simulink model "final"  (R2019b)
settings: Solver=VariableStepAuto  StartTime=0.0  StopTime=70  RelTol=1e-3
undefined symbols (not defined in the file): DiscIntNeverNeededParam, sigbuilder_block
libraries: simulink x2
settings Model: Creator=dayam1  LastModifiedBy=prachurjyas1
settings OptimizationCC: DefaultParameterBehavior=Inlined  EnhancedBackFolding=on  PassReuseOutputArgsThreshold=0  OptimizeBlockOrder=speed  DifferentSizesBufferReuse=on  OptimizationCustomize=off
settings DebuggingCC: SignalInfNanChecking=warning  ParameterTunabilityLossMsg=error  UniqueDataStoreMsg=warning  StrictBusMsg=ErrorOnBusTreatedAsVector
settings SFSimCC: MATLABDynamicMemAlloc=off
settings RTWCC: Description=Generic Real-Time Target  GenerateReport=on  LaunchReport=on
settings CodeAppCC: ForceParamTrailComments=on  OperatorAnnotations=on
settings ConfigComp: CovMetricSettings=dcmwe

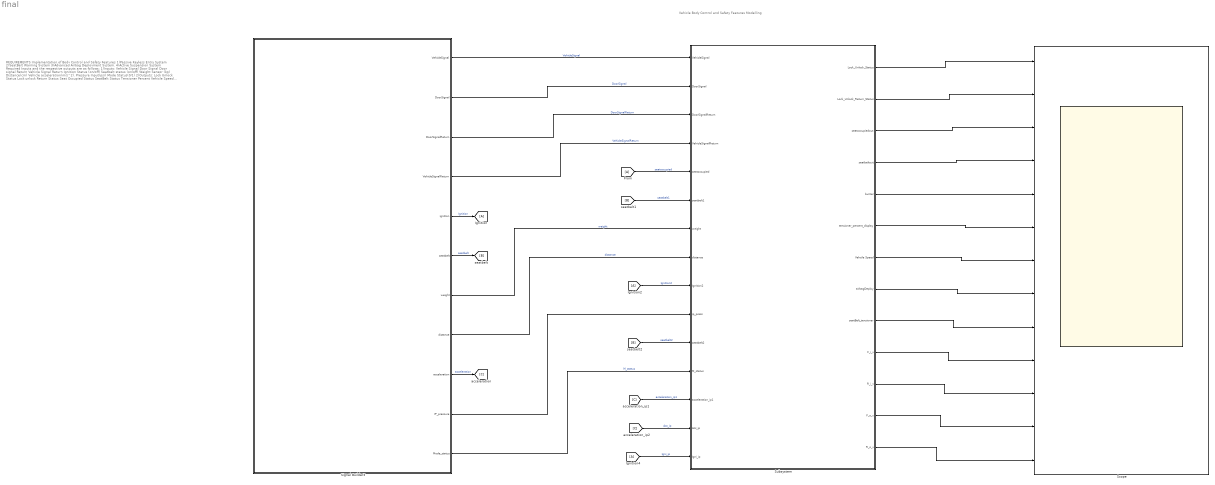
== system final ==
  note: REQUIREMENTS
      |
      | Implementation of Body Control and Safety Features
      | 1)Passive Keyless Entry System
      | 2)SeatBelt Warning System
      | 3)Advanced Airbag Deployment System.
      | 4)Active Suspension System
      |
      | Required Inputs and the respective outputs are as follows:
      | 1)Inputs: Vehicle Signal
      | Door Signal
      | Door signal Return
      | Vehicle Signal Return
      | Ignition Status (on/off)
      | Seatbelt status (on/off)
      | Weight Sensor (kg)
      | Distance(cm)
      | Vehicle acceleration(m/s^2).
      | Pressure Input(psi)
      | Mode Status(0/1)
      |
      | 2)Outputs:
      | Lock Unlock Status
      | Lock unlock Return Status
      | Seat Occupied Status
      | SeatBelt Status
      | Tensioner Percent
      | Vehicle Speed
      | Airbag Deployment
      | Seatbelt tensioner status
      | Steering Status
  note: Vehicle Body Control and Safety Features Modelling
  Scope : Scope  NumInputPorts=13
  Signal Builder3 : Subsystem  Tag=STV Subsys  LoadFcn=sigbuilder_block('load');  StartFcn=sigbuilder_block('start');  StopFcn=sigbuilder_block('stop');  ClipboardFcn=sigbuilder_block('clipboard');  mask(Sigbuilder block){tuvar=[0:10]}
      mask help: Create and generate interchangeable groups of signals whose waveforms are piecewise linear.
      mask init:
      | if ~strcmp(get_param(bdroot(gcbh),'SimulationStatus'),'stopped') tuvar = sigbuilder_block('maskInit'); end
      settings: CopyFcn=sigbuilder_block('copy');  DeleteFcn=sigbuilder_block('delete');  ModelCloseFcn=sigbuilder_block('modelClose');  PreSaveFcn=sigbuilder_block('preSave');  PauseFcn=sigbuilder_block('pause')  ContinueFcn=sigbuilder_block('continue')  NameChangeFcn=sigbuilder_block('namechange');  OpenFcn=sigbuilder_block('open',[6 30 1012.5 447.75 ]);  CloseFcn=sigbuilder_block('close');
      mask Display: plot(0, 0, 100, 100,[2, 2, 32, 32, 2], [68, 8, 8, 68, 68],[32, 2], [38, 38], [32, 19, 2],[53, 60, 44], [32, 17, 17, 2],[16, 16, 31, 31]);txt = getActiveGroup(gcbh);text(2, 100, txt,'verticalAlignment', 'top');
  Subsystem : Subsystem
  wires:
  Signal Builder3/6(seatbelt) -> [B]  "seatbelt"
  Signal Builder3/9(acceleration) -> [C]  "acceleration"
  Signal Builder3/5(ignition) -> [A]  "Ignition"
  [A] -> Subsystem/15(Igni_ip)  "Igni_ip"
  Signal Builder3/1(VehicleSignal) -> Subsystem/1(VehicleSignal)  "VehicleSignal"
  Signal Builder3/2(DoorSignal) -> Subsystem/2(DoorSignal)  "DoorSignal"
  Signal Builder3/3(DoorSignalReturn) -> Subsystem/3(DoorSignalReturn)  "DoorSignalReturn"
  Signal Builder3/4(VehicleSignalReturn) -> Subsystem/4(VehicleSignalReturn)  "VehicleSignalReturn"
  [A] -> Subsystem/5(seatoccupied)  "seatoccupied"
  [B] -> Subsystem/6(seatbelt1)  "seatbelt1"
  Signal Builder3/7(weight) -> Subsystem/7(weight)  "weight"
  Signal Builder3/8(distance) -> Subsystem/8(distance)  "distance"
  [A] -> Subsystem/9(Ignition2)  "Ignition2"
  Signal Builder3/10(IP_pressure) -> Subsystem/10(ip_press)
  [B] -> Subsystem/11(seatbelt2)  "seatbelt2"
  Signal Builder3/11(Mode_status) -> Subsystem/12(M_status)  "M_status"
  [C] -> Subsystem/13(acceleration_ip1)  "acceleration_ip1"
  [C] -> Subsystem/14(Acc_ip)  "Acc_ip"
  Subsystem/1("Lock_Unlock_Status ") -> Scope/1
  Subsystem/2(Lock_Unlock_Return_Status) -> Scope/2
  Subsystem/3(seatoccupiedout) -> Scope/3
  Subsystem/4(seatbeltout) -> Scope/4
  Subsystem/5(buzzer) -> Scope/5
  Subsystem/6(tensioner_percent_display) -> Scope/6
  Subsystem/7(Vehcile Speed) -> Scope/7
  Subsystem/8(airbagDeploy) -> Scope/8
  Subsystem/9(seatBelt_tensioner) -> Scope/9
  Subsystem/10(F_i_v) -> Scope/10
  Subsystem/11(R_i_v) -> Scope/11
  Subsystem/12(F_o_v) -> Scope/12
  Subsystem/13(R_o_v) -> Scope/13

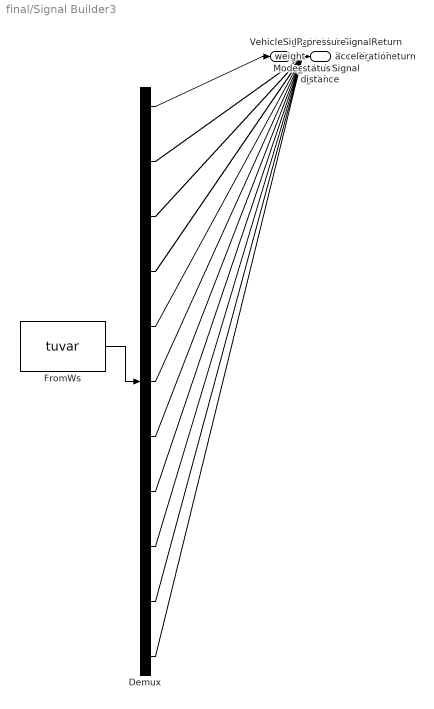
== system final/Signal Builder3 ==
  Demux : Demux  Tag=STV Demux  Outputs=11
  FromWs : FromWorkspace  Tag=STV FromWs  VariableName=tuvar  SampleTime=0
      SigBuilderData=|
      | common.afterFinalStr = 'Extrapolate'
      | common.sampleTime = 0
      | dataSet.timeRange = [0 69]
      | dataSet.name = 'Signal_input'
      | sbobj.Groups.Name = 'Signal_input'
      | sbobj.Groups.Signals(1).Name = 'VehicleSignal'
      | sbobj.Groups.Signals(1).XData = [0 2 10.18 10.18 10.4 10.4 18.94 18.94 20 69]
      | sbobj.Groups.Signals(1).YData = [100 190 558.1 500 500 568 952.3 140 180 180]
      | sbobj.Groups.Signals(2).Name = 'DoorSignal'
      | sbobj.Groups.Signals(2).XData = [0 2 12.26 12.36 12.8 12.8 19.04 19.04 20 69]
      | sbobj.Groups.Signals(2).YData = [0 20 122.6 120 120 128 190.4 -20 -10 -10]
      | sbobj.Groups.Signals(3).Name = 'DoorSignalReturn'
      | sbobj.Groups.Signals(3).XData = [0 18 69]
      | sbobj.Groups.Signals(3).YData = [199.6 0 0]
      | sbobj.Groups.Signals(4).Name = 'VehicleSignalReturn'
      | sbobj.Groups.Signals(4).XData = [0 18 69]
      | sbobj.Groups.Signals(4).YData = [1000 100 100]
      | sbobj.Groups.Signals(5).Name = 'ignition'
      | sbobj.Groups.Signals(5).XData = [0 1 2 3 4 5 6 7 7 8 9 9 10 11 11 12 13 13 14 15 16 17 18 19 20 21 22 23 24 25 26 27 28 29 30 31 31.5 31.9 32.3 32.7 33.1 33.5 33.9 34.3 34.7 35.1 35.5 35.9 36.3 36.7 37.1 37.5 37.9 38.3 39 40 41 42 43 44 45 46 47 48 49 50 51 52 53 54 55 56 57 58 59 60 61 62 63 64 65 66 67 68 69]
      | sbobj.Groups.Signals(5).YData = [0 0 0 1 1 1 1 1 0 0 0 1 1 1 0 0 0 1 1 1 1 1 1 1 1 1 1 1 1 1 1 1 1 1 1 1 0 0 0 0 0 0 0 0 0 0 0 0 0 0 0 0 0 0 0 1 1 1 1 1 1 0 1 1 1 1 0 1 1 0 1 1 1 0 1 1 1 1 1 1 1 1 1 1 0]
      | sbobj.Groups.Signals(6).Name = 'seatbelt'
      | sbobj.Groups.Signals(6).XData = [0 1 2 3 3 4 4 5 6 7 7 8 9 10 11 12 13 13 14 15 16 17 18 18 19 20 21 22 23 24 25 26 27 28 29 30 31 31 31.5 31.9 32.3 32.7 33.1 33.5 33.9 34.3 34.7 35.1 35.5 35.9 36.3 36.7 37.1 37.5 37.9 38.3 39 40 40 41 42 43 44 45 46 47 48 49 50 50 51 52 53 54 55 56 57 58 59 60 60 61 62 63 64 65 66 67 68 69]
      | sbobj.Groups.Signals(6).YData = [0 0 0 0 1 1 0 0 0 0 1 1 1 1 1 1 1 0 0 0 0 0 0 1 1 1 1 1 1 1 1 1 1 1 1 1 1 0 0 0 1 1 1 1 1 1 1 1 1 1 1 1 1 1 1 1 1 1 0 0 1 1 1 1 1 1 1 1 1 0 0 1 1 1 1 1 1 1 1 1 0 0 1 1 1 1 1 1 1 1]
      | sbobj.Groups.Signals(7).Name = 'weight'
      | sbobj.Groups.Signals(7).XData = [0 1 1 2 2 3 3 4 4 5 5 6 6 7 7 8 8 9 9 10 10 11 11 12 12 13 13 14 14 15 15 16 16 17 17 18 18 19 19 20 20 21 21 22 23 24 24 25 25 26 26 27 27 28 28 29 29 30 30 31 31 31.5 31.9 32.3 32.7 33.1 33.5 33.9 34.3 34.7 35.1 35.5 35.9 36.3 36.7 37.1 37.5 37.9 38.3 39 40 41 42 43 44 45 46 47 48 49 50 51 52 52 53 53 54 55 56 57 58 58 59 60 60 61 62 63 63 64 64 65 65 66 66 67 67 68 68 69]
      | sbobj.Groups.Signals(7).YData = [78 78 68 66 55 55 87 87 43 43 30 30 20 20 10 10 70 70 88 88 99 99 66 66 54 54 34 34 44 44 89 89 86 86 10 10 54 54 44 44 99 99 75 106 106 50 25 25 33 33 26 26 57 57 78 78 57 57 78 78 86 10 10 54 54 44 44 99 99 75 106 106 106 106 50 25 25 33 33 66 55 87 43 30 20 10 70 88 99 66 54 34 44 78 78 86 10 54 44 99 75 106 106 106 50 25 33 66 78 86 10 10 54 54 44 44 99 99 75 106]
      | sbobj.Groups.Signals(8).Name = 'distance'
      | sbobj.Groups.Signals(8).XData = [0 1 2 3 4 5 6 7 8 9 10 11 12 13 14 15 16 17 18 19 20 21 22 23 24 25 26 27 28 29 30 31 31 31.5 31.9 32.3 32.7 33.1 33.5 33.9 34.3 34.7 35.1 35.5 35.9 36.3 36.7 37.1 37.5 37.9 38.3 39 40 40 41 41 42 42 43 43 44 44 45 45 46 46 47 47 48 48 49 49 50 51 52 53 54 55 56 57 58 59 60 60 61 61 62 62 63 63 64 64 65 65 66 66 67 67 68 68 69]
      | sbobj.Groups.Signals(8).YData = [21 22 24 10 18 23 29 50 23 16 13 21 22 19 14 24 15 19 11 22 17 22 24 10 18 23 29 50 23 50 23 23 19 19 11 11 22 22 17 17 22 22 24 24 10 10 18 18 23 23 29 17 17 22 22 24 24 10 10 18 18 23 23 29 29 50 50 23 23 50 50 23 23 19 11 22 17 22 24 10 18 23 29 17 17 22 22 24 24 10 10 18 18 23 23 29 29 50 50 23 23]
      | sbobj.Groups.Signals(9).Name = 'acceleration'
      | sbobj.Groups.Signals(9).XData = [0 1 2 3 4 5 6 7 8 9 10 11 12 13 14 15 16 17 18 19 20 21 22 23 24 25 26 27 28 29 30 31 31 31.5 31.9 32.3 32.7 33.1 33.5 33.9 34.3 34.7 35.1 35.5 35.9 36.3 36.7 37.1 37.5 37.9 38.3 39 40 41 42 43 44 45 46 47 48 49 50 51 52 53 54 55 56 57 58 59 60 61 62 63 64 65 66 67 68 69]
      | sbobj.Groups.Signals(9).YData = [9 12 45 54 67 12 47 34 67 23 89 23 52 9 76 13 67 34 90 28 49 12 45 54 67 12 47 34 67 34 67 67 34 34 90 90 90 90 90 90 90 90 90 45 54 54 67 67 12 12 47 12 45 54 67 20 50 34 67 23 89 23 52 76 50 13 67 45 14 88 49 42 45 24 67 12 99 34 67 50 99 9]
      | sbobj.Groups.Signals(10).Name = 'IP_pressure'
      | sbobj.Groups.Signals(10).XData = [0 1 2 3 4 5 6 7 8 9 10 11 12 13 14 15 16 17 18 19 20 21 22 23 24 25 26 27 28 29 30 31 31 31.5 31.9 32.3 32.7 33.1 33.5 33.9 34.3 34.7 35.1 35.5 35.9 36.3 36.7 37.1 37.5 37.9 38.3 39 40 41 42 43 44 45 46 47 48 49 50 51 52 53 54 55 56 57 58 59 60 61 62 63 64 65 66 67 68 69]
      | sbobj.Groups.Signals(10).YData = [-100 -80 60 45 65 100 76 23 98 45 119 102 99 66 34 56 22 97 67 9 78 -80 60 45 65 100 76 23 98 23 0 0 97 97 67 67 9 9 78 78 -80 -80 60 60 45 45 65 65 100 100 76 -50 -10 10 30 50 50 100 110 100 40 80 140 50 50 15 17 100 100 100 88 100 50 50 44 66 50 50 100 100 50 -100]
      | sbobj.Groups.Signals(11).Name = 'Mode_status'
      | sbobj.Groups.Signals(11).XData = [0 1 2 2 3 4 5 6 7 7 8 9 9 10 11 11 12 13 13 14 15 16 17 18 19 20 21 22 22 23 24 25 26 27 27 28 29 30 31 31.5 31.9 32.3 32.7 33.1 33.5 33.9 34.3 34.7 35.1 35.5 35.9 36.3 36.7 37.1 37.5 37.9 38.3 39 40 41 42 43 44 45 46 47 48 49 50 51 52 53 54 55 56 57 58 59 60 61 62 63 64 65 66 67 68 69]
      | sbobj.Groups.Signals(11).YData = [0 0 0 1 1 1 1 1 1 0 0 0 1 1 1 0 0 0 1 1 1 1 1 1 1 1 0 0 1 1 1 1 1 1 0 0 1 1 1 1 1 1 1 1 1 1 0 0 0 1 1 1 1 1 1 1 1 0 1 1 1 0 0 1 1 1 0 0 0 0 0 0 0 1 1 1 0 1 0 0 0 0 0 0 1 1 0 0]
      | sbobj.Groups.TimeRange = [0 69]
  VehicleSignal : Outport  Tag=STV Outport  VectorParamsAs1DForOutWhenUnconnected=off
  DoorSignal : Outport  Tag=STV Outport  Port=2
  DoorSignalReturn : Outport  Tag=STV Outport  Port=3
  VehicleSignalReturn : Outport  Tag=STV Outport  Port=4
  ignition : Outport  Tag=STV Outport  Port=5
  seatbelt : Outport  Tag=STV Outport  Port=6
  weight : Outport  Tag=STV Outport  Port=7
  distance : Outport  Tag=STV Outport  Port=8
  acceleration : Outport  Tag=STV Outport  Port=9
  IP_pressure : Outport  Tag=STV Outport  Port=10
  Mode_status : Outport  Tag=STV Outport  Port=11
  wires:
  FromWs/1 -> Demux/1
  Demux/1 -> VehicleSignal/1
  Demux/2 -> DoorSignal/1
  Demux/3 -> DoorSignalReturn/1
  Demux/4 -> VehicleSignalReturn/1
  Demux/5 -> ignition/1
  Demux/6 -> seatbelt/1
  Demux/7 -> weight/1
  Demux/8 -> distance/1
  Demux/9 -> acceleration/1
  Demux/10 -> IP_pressure/1
  Demux/11 -> Mode_status/1

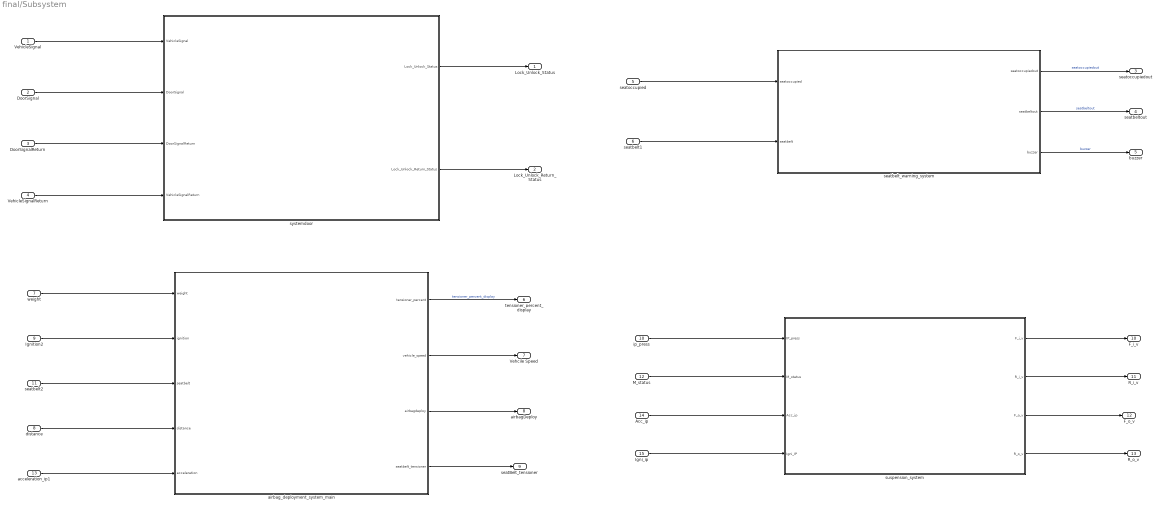
== system final/Subsystem ==
  VehicleSignal : Inport
  DoorSignal : Inport  Port=2
  DoorSignalReturn : Inport  Port=3
  VehicleSignalReturn : Inport  Port=4
  seatoccupied : Inport  Port=5
  seatbelt1 : Inport  Port=6
  weight : Inport  Port=7
  distance : Inport  Port=8
  Ignition2 : Inport  Port=9
  ip_press : Inport  Port=10
  seatbelt2 : Inport  Port=11
  M_status : Inport  Port=12
  acceleration_ip1 : Inport  Port=13
  Acc_ip : Inport  Port=14
  Igni_ip : Inport  Port=15
  airbag_deployment_system_main : Subsystem
  seatbelt_warning_system : Subsystem
  suspension_system : Subsystem
  systemdoor : Subsystem
  "Lock_Unlock_Status " : Outport
  Lock_Unlock_Return_Status : Outport  Port=2
  seatoccupiedout : Outport  Port=3
  seatbeltout : Outport  Port=4
  buzzer : Outport  Port=5
  tensioner_percent_display : Outport  Port=6
  Vehcile Speed : Outport  Port=7
  airbagDeploy : Outport  Port=8
  seatBelt_tensioner : Outport  Port=9
  F_i_v : Outport  Port=10
  R_i_v : Outport  Port=11
  F_o_v : Outport  Port=12
  R_o_v : Outport  Port=13
  wires:
  distance/1 -> airbag_deployment_system_main/4(distance)
  airbag_deployment_system_main/4(seatbelt_tensioner) -> seatBelt_tensioner/1
  Ignition2/1 -> airbag_deployment_system_main/2(ignition)
  seatoccupied/1 -> seatbelt_warning_system/1(seatoccupied)
  acceleration_ip1/1 -> airbag_deployment_system_main/5(acceleration)
  systemdoor/1(Lock_Unlock_Status) -> "Lock_Unlock_Status "/1
  airbag_deployment_system_main/2(vehicle_speed) -> Vehcile Speed/1
  airbag_deployment_system_main/3(airbagdeploy) -> airbagDeploy/1
  DoorSignalReturn/1 -> systemdoor/3(DoorSignalReturn)
  airbag_deployment_system_main/1(tensioner_percent) -> tensioner_percent_display/1  "tensioner_percent_display"
  VehicleSignal/1 -> systemdoor/1(VehicleSignal)
  seatbelt2/1 -> airbag_deployment_system_main/3(seatbelt)
  seatbelt1/1 -> seatbelt_warning_system/2(seatbelt)
  systemdoor/2(Lock_Unlock_Return_Status) -> Lock_Unlock_Return_Status/1
  DoorSignal/1 -> systemdoor/2(DoorSignal)
  VehicleSignalReturn/1 -> systemdoor/4(VehicleSignalReturn)
  seatbelt_warning_system/2(seatbeltout) -> seatbeltout/1  "seatbeltout"
  seatbelt_warning_system/3(buzzer) -> buzzer/1  "buzzer"
  weight/1 -> airbag_deployment_system_main/1(weight)
  seatbelt_warning_system/1(seatoccupiedout) -> seatoccupiedout/1  "seatoccupiedout"
  ip_press/1 -> suspension_system/1(IP_press)
  M_status/1 -> suspension_system/2(M_status)
  Acc_ip/1 -> suspension_system/3(Acc_ip)
  Igni_ip/1 -> suspension_system/4(Igni_IP)
  suspension_system/1(F_i_v) -> F_i_v/1
  suspension_system/2(R_i_v) -> R_i_v/1
  suspension_system/3(F_o_v) -> F_o_v/1
  suspension_system/4(R_o_v) -> R_o_v/1

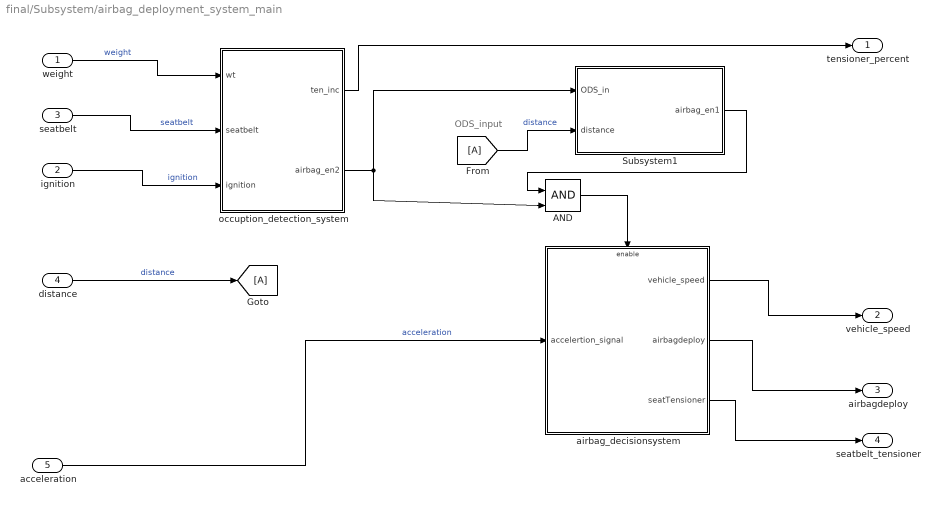
== system final/Subsystem/airbag_deployment_system_main ==
  note: ODS_input
  weight : Inport
  ignition : Inport  Port=2
  seatbelt : Inport  Port=3
  distance : Inport  Port=4
  acceleration : Inport  Port=5
  AND : Logic  IconShape=distinctive  AllPortsSameDT=off  OutDataTypeStr=boolean
  Subsystem1 : Subsystem
  airbag_decisionsystem : Subsystem
  occuption_detection_system : Subsystem
  tensioner_percent : Outport
  vehicle_speed : Outport  Port=2
  airbagdeploy : Outport  Port=3
  seatbelt_tensioner : Outport  Port=4
  wires:
  occuption_detection_system/2(airbag_en2) -> Subsystem1/1(ODS_in), AND/2
  distance/1 -> [A]  "distance"
  acceleration/1 -> airbag_decisionsystem/1(accelertion_signal)  "acceleration"
  airbag_decisionsystem/2(airbagdeploy) -> airbagdeploy/1
  [A] -> Subsystem1/2(distance)  "distance"
  airbag_decisionsystem/3(seatTensioner) -> seatbelt_tensioner/1
  airbag_decisionsystem/1(vehicle_speed) -> vehicle_speed/1
  occuption_detection_system/1(ten_inc) -> tensioner_percent/1
  weight/1 -> occuption_detection_system/1(wt)  "weight"
  ignition/1 -> occuption_detection_system/3(ignition)  "ignition"
  seatbelt/1 -> occuption_detection_system/2(seatbelt)  "seatbelt"
  Subsystem1/1(airbag_en1) -> AND/1
  AND/1 -> airbag_decisionsystem/Enable

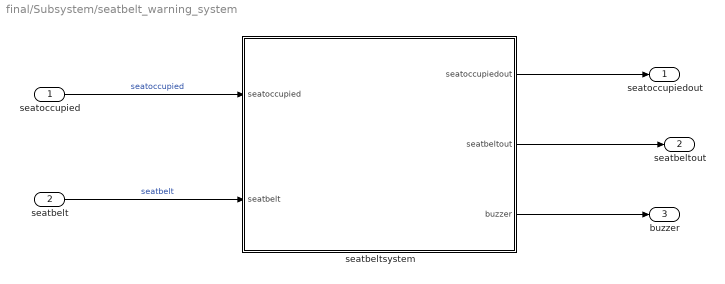
== system final/Subsystem/seatbelt_warning_system ==
  seatoccupied : Inport
  seatbelt : Inport  Port=2
  seatbeltsystem : Stateflow chart  TreatAsAtomicUnit=on
  seatoccupiedout : Outport
  seatbeltout : Outport  Port=2
  buzzer : Outport  Port=3
  wires:
  seatoccupied/1 -> seatbeltsystem/1(seatoccupied)  "seatoccupied"
  seatbeltsystem/2(seatbeltout) -> seatbeltout/1
  seatbelt/1 -> seatbeltsystem/2(seatbelt)  "seatbelt"
  seatbeltsystem/3(buzzer) -> buzzer/1
  seatbeltsystem/1(seatoccupiedout) -> seatoccupiedout/1

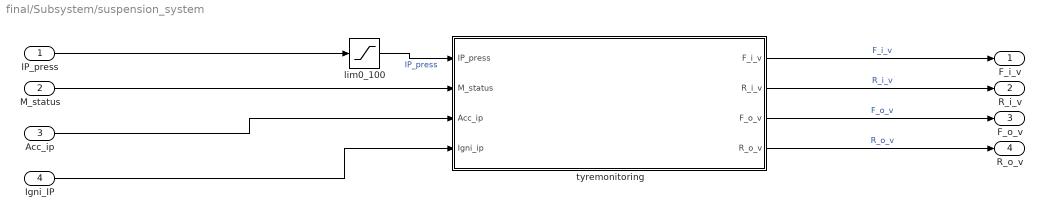
== system final/Subsystem/suspension_system ==
  IP_press : Inport
  M_status : Inport  Port=2
  Acc_ip : Inport  Port=3
  Igni_IP : Inport  Port=4
  lim0_100 : Saturate  UpperLimit=120  LowerLimit=0
      settings: AttributesFormatString=|
      | %<LowerLimit>=0
      | %<UpperLimit>=120
  tyremonitoring : Stateflow chart  BlockKeywords=__PRM__SERIALIZED__DATA__:Stateflow Chart,Stateflow Diagram  TreatAsAtomicUnit=on
  F_i_v : Outport
  R_i_v : Outport  Port=2
  F_o_v : Outport  Port=3
  R_o_v : Outport  Port=4
  wires:
  tyremonitoring/2(R_i_v) -> R_i_v/1  "R_i_v"
  tyremonitoring/4(R_o_v) -> R_o_v/1  "R_o_v"
  tyremonitoring/1(F_i_v) -> F_i_v/1  "F_i_v"
  lim0_100/1 -> tyremonitoring/1(IP_press)  "IP_press"
  Acc_ip/1 -> tyremonitoring/3(Acc_ip)
  M_status/1 -> tyremonitoring/2(M_status)
  tyremonitoring/3(F_o_v) -> F_o_v/1  "F_o_v"
  Igni_IP/1 -> tyremonitoring/4(Igni_ip)
  IP_press/1 -> lim0_100/1

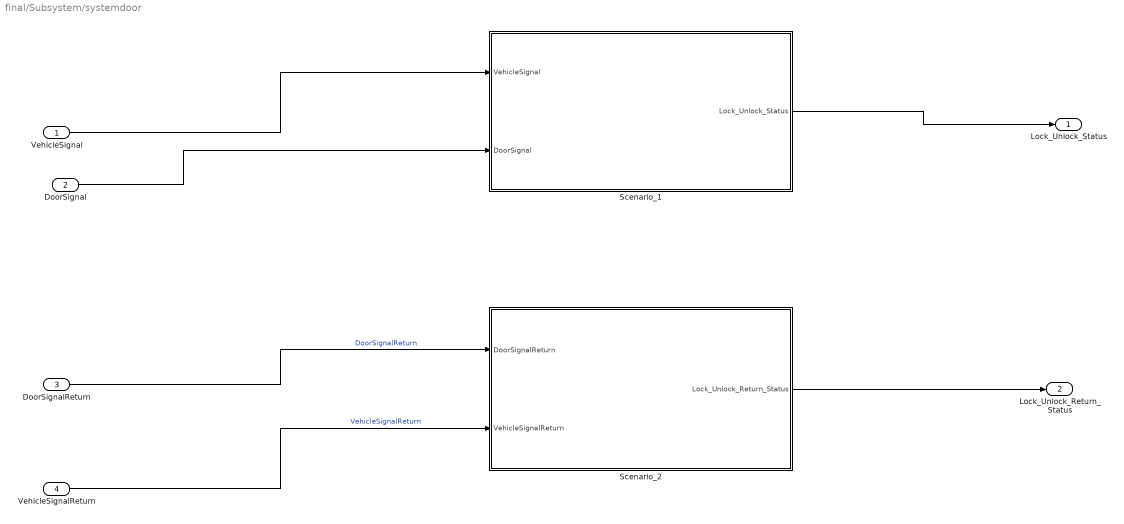
== system final/Subsystem/systemdoor ==
  VehicleSignal : Inport
  DoorSignal : Inport  Port=2
  DoorSignalReturn : Inport  Port=3
  VehicleSignalReturn : Inport  Port=4
  Scenario_1 : Stateflow chart  TreatAsAtomicUnit=on
  Scenario_2 : Stateflow chart  TreatAsAtomicUnit=on
  Lock_Unlock_Status : Outport
  Lock_Unlock_Return_Status : Outport  Port=2
  wires:
  DoorSignal/1 -> Scenario_1/2(DoorSignal)
  VehicleSignal/1 -> Scenario_1/1(VehicleSignal)
  DoorSignalReturn/1 -> Scenario_2/1(DoorSignalReturn)  "DoorSignalReturn"
  Scenario_1/1(Lock_Unlock_Status) -> Lock_Unlock_Status/1
  Scenario_2/1(Lock_Unlock_Return_Status) -> Lock_Unlock_Return_Status/1
  VehicleSignalReturn/1 -> Scenario_2/2(VehicleSignalReturn)  "VehicleSignalReturn"

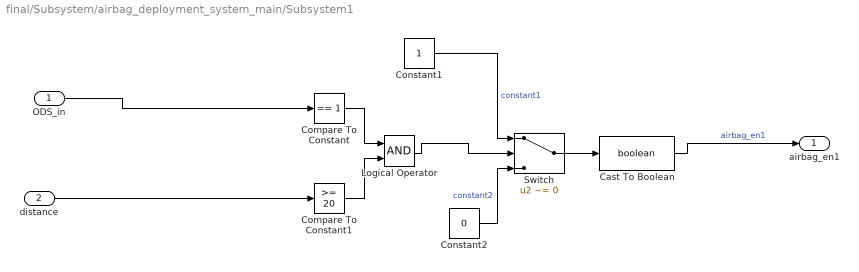
== system final/Subsystem/airbag_deployment_system_main/Subsystem1 ==
  ODS_in : Inport
  distance : Inport  Port=2
  Cast To Boolean : DataTypeConversion  OutDataTypeStr=boolean
  Compare To Constant : simulink/Logic and Bit Operations/Compare To Constant  relop===  const=1  OutDataTypeStr=boolean
  Compare To Constant1 : simulink/Logic and Bit Operations/Compare To Constant  relop=>=  const=20  OutDataTypeStr=boolean
  Constant1 : Constant
  Constant2 : Constant  Value=0
  Logical Operator : Logic  AllPortsSameDT=off  OutDataTypeStr=boolean
  Switch : Switch  Criteria=u2 ~= 0
  airbag_en1 : Outport  OutDataTypeStr=boolean
  wires:
  distance/1 -> Compare To Constant1/1
  Compare To Constant1/1 -> Logical Operator/2
  ODS_in/1 -> Compare To Constant/1
  Logical Operator/1 -> Switch/2
  Constant2/1 -> Switch/3  "constant2"
  Constant1/1 -> Switch/1  "constant1"
  Compare To Constant/1 -> Logical Operator/1
  Switch/1 -> Cast To Boolean/1
  Cast To Boolean/1 -> airbag_en1/1  "airbag_en1"

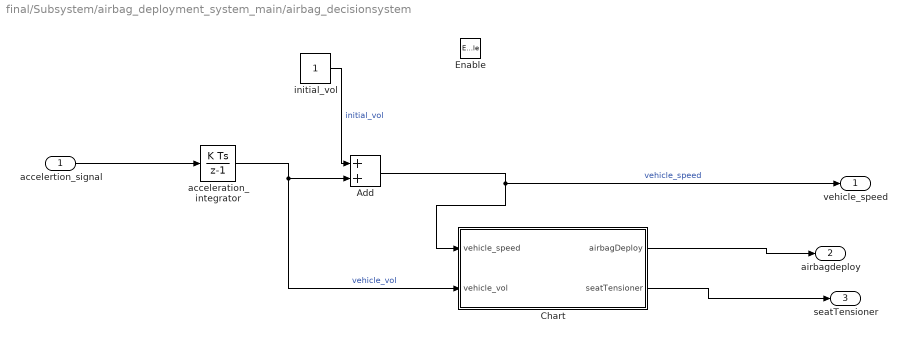
== system final/Subsystem/airbag_deployment_system_main/airbag_decisionsystem ==
  accelertion_signal : Inport
  Enable : EnablePort
  Add : Sum
  Chart : Stateflow chart  TreatAsAtomicUnit=on
  acceleration_integrator : DiscreteIntegrator  SampleTime=-1  ICPrevOutput=DiscIntNeverNeededParam  ICPrevScaledInput=DiscIntNeverNeededParam
  initial_vol : Constant
  vehicle_speed : Outport
  airbagdeploy : Outport  Port=2
  seatTensioner : Outport  Port=3
  wires:
  Add/1 -> vehicle_speed/1, Chart/1(vehicle_speed)  "vehicle_speed"
  Chart/1(airbagDeploy) -> airbagdeploy/1
  Chart/2(seatTensioner) -> seatTensioner/1
  initial_vol/1 -> Add/1  "initial_vol"
  accelertion_signal/1 -> acceleration_integrator/1
  acceleration_integrator/1 -> Add/2, Chart/2(vehicle_vol)  "vehicle_vol"

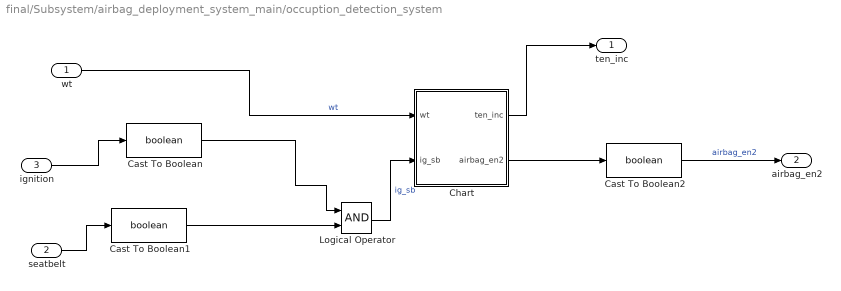
== system final/Subsystem/airbag_deployment_system_main/occuption_detection_system ==
  wt : Inport
  seatbelt : Inport  Port=2
  ignition : Inport  Port=3
  Cast To Boolean : DataTypeConversion  OutDataTypeStr=boolean
  Cast To Boolean1 : DataTypeConversion  OutDataTypeStr=boolean
  Cast To Boolean2 : DataTypeConversion  OutDataTypeStr=boolean
  Chart : Stateflow chart  TreatAsAtomicUnit=on
  Logical Operator : Logic  AllPortsSameDT=off  OutDataTypeStr=boolean
  ten_inc : Outport
  airbag_en2 : Outport  Port=2
  wires:
  Logical Operator/1 -> Chart/2(ig_sb)  "ig_sb"
  Cast To Boolean1/1 -> Logical Operator/2
  Cast To Boolean/1 -> Logical Operator/1
  Chart/1(ten_inc) -> ten_inc/1
  ignition/1 -> Cast To Boolean/1
  seatbelt/1 -> Cast To Boolean1/1
  Chart/2(airbag_en2) -> Cast To Boolean2/1
  Cast To Boolean2/1 -> airbag_en2/1  "airbag_en2"
  wt/1 -> Chart/1(wt)  "wt"

== stateflow chart final/Subsystem/seatbelt_warning_system/seatbeltsystem ==
  state Idle_state
    en:
    seatoccupiedout=0;
    buzzer=0;
    seatbeltout=0;
  state Seatoccupied
    en:
    seatoccupiedout=1;
  state Buzzer
    en:
    seatbeltout=0;
    buzzer=1;
    disp('buzzer on');
  state SeatbeltOn
    en:
    seatbeltout=1;
    buzzer=0;
  (default) -> Idle_state
  Idle_state -> Seatoccupied : [seatoccupied==1]
  SeatbeltOn -> Idle_state : [seatoccupied==0]
  Buzzer -> Idle_state [order 1] : [seatoccupied==0]
  Seatoccupied -> Buzzer [order 2] : [seatbelt==0]
  Seatoccupied -> SeatbeltOn [order 1] : [seatbelt==1]
  Buzzer -> SeatbeltOn [order 2] : [seatbelt==1]
  data: seatoccupied input; seatbelt input; seatoccupiedout output; seatbeltout output; buzzer output; c local

== stateflow chart final/Subsystem/airbag_deployment_system_main/airbag_decisionsystem/Chart ==
  state normalState
    en, du:
    airbagDeploy=0;
    seatTensioner=0;
  state standbyState
    en, du:
    airbagDeploy=0;
    seatTensioner=1;
  state fireState
    en, du:
    airbagDeploy=1;
    seatTensioner=1;
  (default) -> normalState
  standbyState -> fireState [order 1] : [vehicle_speed>=22.54]
  normalState -> standbyState : [vehicle_vol>=Vth]
  standbyState -> fireState [order 3] : [12.88<vehicle_speed<22.54]
  fireState -> standbyState : [vehicle_speed<12.88]
  standbyState -> normalState [order 2] : [vehicle_vol<Vth]
  data: Vth local =1; vehicle_speed input; vehicle_vol input; airbagDeploy output; seatTensioner output

== stateflow chart final/Subsystem/airbag_deployment_system_main/occuption_detection_system/Chart ==
  state systemOn
    exit:
    airbag_en2=1;
    (default) -> (junction 15) : % tension adjuster
    (junction 15) -> (junction 16) [order 1] : [wt>=75.0 && wt<=100.0]
    (junction 15) -> (junction 17) [order 2]
    (junction 16) -> (junction 24) : {ten_inc=10.0+Tini;}
    (junction 17) -> (junction 18) [order 1] : [wt>=50.0 && wt<=75.0]
    (junction 17) -> (junction 19) [order 2]
    (junction 18) -> (junction 23) : {ten_inc=20.0+Tini;}
    (junction 19) -> (junction 20) [order 1] : [wt>=25.0 && wt<=50.0]
    (junction 19) -> (junction 21) [order 2] : {ten_inc=Tini;}
    (junction 20) -> (junction 22) : {ten_inc=30.0+Tini;}
    (junction 22) -> (junction 21)
    (junction 23) -> (junction 22)
    (junction 24) -> (junction 23)
    (junction 21) -> (junction 25)
  state systemOff
    exit:
    airbag_en2=0;
  (default) -> systemOn
  systemOn -> systemOff : [ig_sb==1.0]
  systemOff -> systemOn : [ig_sb==0]
  data: wt input; Tini local =5; ten_inc output; ig_sb input; airbag_en2 output

== stateflow chart final/Subsystem/systemdoor/Scenario_1 ==
  settings: updateMethod=DISCRETE  sampleTime=0.01
  note: Scenario 1: When user is moving away from the source
  state VehicleSensor [parallel]
    settings: executionOrder=2
    state Active
      en:
      VehicleActive  =  1;
    state Inactive
      en:
      VehicleActive  =  0;
      en:
      count  =  100;
      du:
      count  =  count + 50;
    (default) -> VehicleSensor.Active
    VehicleSensor.Inactive -> VehicleSensor.Active [order 2] : [count >= 750]
    VehicleSensor.Active -> VehicleSensor.Inactive : [VehicleSignal >= 100]
    VehicleSensor.Inactive -> VehicleSensor.Inactive [order 1] : [VehicleSignal > 100]
  note: %% Vehicle Sensor
      | % When the signal value goes from 100 to 750, the Vehicle state activates
      | % When it reaches the 750 count, the door locks
  state DoorStatus [parallel]
    settings: executionOrder=3
    (default) -> (junction 20)
    DoorStatus -> (junction 20)
    (junction 20) -> (junction 22) [order 1] : [VehicleActive && DoorActive == 1 ]
    (junction 20) -> (junction 30) [order 2]
    (junction 22) -> (junction 24) : {Lock_Unlock_Status = 1;}
    (junction 30) -> (junction 32) [order 1] : [VehicleActive]
    (junction 30) -> (junction 38) [order 2]
    (junction 32) -> (junction 34) : {Lock_Unlock_Status = 2;}
    (junction 38) -> (junction 40) [order 1] : [DoorActive]
    (junction 38) -> (junction 26) [order 2] : {Lock_Unlock_Status = 0;}
    (junction 40) -> (junction 36) : {Lock_Unlock_Status = 3;}
    (junction 36) -> (junction 26)
    (junction 34) -> (junction 36)
    (junction 24) -> (junction 34)
  state DoorSensor [parallel]
    settings: executionOrder=1
    state Active
      en:
      DoorActive  =  1;
    state Inactive
      en:
      DoorActive = 0;
      en:
      count = 1;
      du:
      count = count + 10;
    (default) -> DoorSensor.Active
    DoorSensor.Inactive -> DoorSensor.Active [order 2] : [count >=100]
    DoorSensor.Active -> DoorSensor.Inactive : [DoorSignal >= 0]
    DoorSensor.Inactive -> DoorSensor.Inactive [order 1] : [DoorSignal > 0]
  note: %% Door Sensor
      | % When the signal value goes from 0 to 100, the Door state activates
      | % When it reaches the 100 count, the still stays the same
  note: %% Door Status
      | % When both the states are active, only then the output status is given.
      | % Otherwise the door remains open
  data: count local; count local; Lock_Unlock_Status output double; VehicleSignal input; DoorSignal input; VehicleActive local; DoorActive local

== stateflow chart final/Subsystem/systemdoor/Scenario_2 ==
  settings: updateMethod=DISCRETE  sampleTime=0.01
  note: Scenario 2: When user is moving towards source
  state VehicleSensor [parallel]
    settings: executionOrder=2
    state Active
      en:
      VehicleRange  =  0;
    state Inactive
      en:
      VehicleRange  =  1;
      en:
      count  =  750;
      du:
      count  =  count - 50;
    (default) -> VehicleSensor.Active
    VehicleSensor.Inactive -> VehicleSensor.Active [order 2] : [count > 100]
    VehicleSensor.Active -> VehicleSensor.Inactive : [VehicleSignalReturn <= 750]
    VehicleSensor.Inactive -> VehicleSensor.Inactive [order 1] : [VehicleSignalReturn < 750]
  state DoorStatus [parallel]
    settings: executionOrder=3
    (default) -> (junction 20)
    DoorStatus -> (junction 20)
    (junction 20) -> (junction 22) [order 1] : [VehicleRange && DoorRange]
    (junction 20) -> (junction 30) [order 2]
    (junction 22) -> (junction 24) : {Lock_Unlock_Return_Status = 1;}
    (junction 30) -> (junction 32) [order 1] : [VehicleRange]
    (junction 30) -> (junction 38) [order 2]
    (junction 32) -> (junction 34) : {Lock_Unlock_Return_Status = 2;}
    (junction 38) -> (junction 40) [order 1] : [DoorRange]
    (junction 38) -> (junction 26) [order 2] : {Lock_Unlock_Return_Status = 0;}
    (junction 40) -> (junction 36) : {Lock_Unlock_Return_Status = 3;}
    (junction 36) -> (junction 26)
    (junction 34) -> (junction 36)
    (junction 24) -> (junction 34)
  note: %% Vehicle Sensor
      | % When the signal value goes from 750 to 100, the Vehicle state activates
      | % When it reaches the 100 count, the door locks
  state DoorSensor [parallel]
    settings: executionOrder=1
    state Active
      en:
      DoorRange =  0;
    state Inactive
      en:
      DoorRange = 1;
      en:
      count = 100;
      du:
      count = count - 10;
    (default) -> DoorSensor.Active
    DoorSensor.Inactive -> DoorSensor.Active [order 2] : [count > 0]
    DoorSensor.Active -> DoorSensor.Inactive : [DoorSignalReturn <= 100]
    DoorSensor.Inactive -> DoorSensor.Inactive [order 1] : [DoorSignalReturn < 100]
  note: %% Door Sensor
      | % When the signal value goes from 100 to 0, the Door state activates
      | % When it reaches the 0 count, the door unlocks
  note: %% Door Status
      | % When both the states are active, only then the output status is given.
      | % Otherwise the door remains closed
  data: count local; count local; DoorSignalReturn input; VehicleRange local; DoorRange local; VehicleSignalReturn input; Lock_Unlock_Return_Status output

== stateflow chart final/Subsystem/suspension_system/tyremonitoring ==
  state Ignition_OFF
    en:
    F_o_v =0;
    R_o_v=0;
    F_i_v =0;
    R_i_v=0;
  state Ignition_ON
    state City_mode
      (junction 21) -> (junction 25) [order 3] : [IP_press==50]
      City_mode -> (junction 21) [order 1]
      (junction 21) -> (junction 25) [order 1] : [IP_press<50]{F_i_v=1;R_i_v=1;F_o_v=0;R_o_v=0}
      (junction 21) -> (junction 25) [order 2] : [IP_press>50]{F_o_v=1;R_o_v=1;F_i_v=0;R_i_v=0}
      (junction 25) -> (junction 35) [order 1] : [IP_press==50 && Acc_ip >30&&Acc_ip<60]
      (junction 25) -> (junction 40) [order 2] : [IP_press==50 && Acc_ip>60]
      (junction 25) -> (junction 45) [order 3] : [IP_press==50 && Acc_ip <30]
      (junction 25) -> (junction 24) [order 4]
      (junction 35) -> (junction 36) : {F_i_v=0;R_i_v=0}
      (junction 40) -> (junction 41) : {F_i_v=0;R_i_v=1}
      (junction 45) -> (junction 46) : {F_i_v=1;R_i_v=0}
      (junction 46) -> (junction 24) : {F_o_v=0;R_o_v=0}
      (junction 41) -> (junction 24) : {F_o_v=0;R_o_v=0}
      (junction 36) -> (junction 24) : {F_o_v=0;R_o_v=0}
    state HIghway_mode
      (junction 73) -> (junction 68) [order 3] : [IP_press==100]
      HIghway_mode -> (junction 73) [order 1]
      (junction 73) -> (junction 68) [order 1] : [IP_press<100]{F_i_v=1;R_i_v=1;F_o_v=0;R_o_v=0}
      (junction 73) -> (junction 68) [order 2] : [IP_press>100]{F_o_v=1;R_o_v=1;F_i_v=0;R_i_v=0}
      (junction 68) -> (junction 55) [order 1] : [IP_press==100 && Acc_ip >30&&Acc_ip<60]
      (junction 68) -> (junction 63) [order 2] : [IP_press==100 && Acc_ip >60]
      (junction 68) -> (junction 60) [order 3] : [IP_press==100 && Acc_ip<30]
      (junction 68) -> (junction 69) [order 4]
      (junction 55) -> (junction 53) : {F_i_v=0;R_i_v=0}
      (junction 63) -> (junction 57) : {F_i_v=0;R_i_v=1}
      (junction 60) -> (junction 64) : {F_i_v=1;R_i_v=0}
      (junction 64) -> (junction 69) : {F_o_v=0;R_o_v=0}
      (junction 57) -> (junction 69) : {F_o_v=0;R_o_v=0}
      (junction 53) -> (junction 69) : {F_o_v=0;R_o_v=0}
    (default) -> City_mode
    HIghway_mode -> City_mode [order 1] : [M_status==0]
    City_mode -> HIghway_mode [order 1] : [M_status==1]
  (default) -> Ignition_OFF
  Ignition_OFF -> Ignition_ON : [Igni_ip ==1]
  Ignition_ON -> Ignition_OFF : [Igni_ip==0]
  data: IP_press input; M_status input; Acc_ip input; Igni_ip input; F_i_v output; R_i_v output; F_o_v output; R_o_v output
